simulink model "Modello_Irb1300_R2022a"  (R2022a)
settings: Solver=VariableStepAuto  StartTime=0.0  StopTime=56.0  RelTol=1e-3
undefined symbols (not defined in the file or in its folder): DiscIntNeverNeededParam
libraries: vrlib x3, simulink x1
(part 2 of 2)

== matlab function Modello_Irb1300_R2022a/MATLAB Function6 ==
  data: O_d input; R_error output; R_a input
function R_error = Orientation(O_d,R_a)
% R_a, è la matrice di rotazione ottenuta dalla posa in retroazione 

%R_iniziale, questa matrice è la matrice iniziale (orientzione assoluta) 
%che permette di riferire gli angoli di eulero alla orientazione relativa dell'end effector
R_iniziale = [
    0.0000    0.0000    1.0000 ;
    1.0000         0    0.0000 ;
         0    1.0000    0.0000 ];
% Angolipi di Eulero in radianti
theta = O_d(1);  % Rotazione attorno all'asse x 
phi = O_d(2);    % Rotazione attorno all'asse y 
psi = O_d(3);    % Rotazione attorno all'asse z (psi = 0° otteniamo una rotazione dell'end effector di 90°)

% Matrici di rotazione elementari
R_x = [
      1, 0, 0;
      0, cos(theta), -sin(theta);
      0, sin(theta), cos(theta)
];

R_y = [
    cos(phi), 0, sin(phi);
    0, 1, 0;
    -sin(phi), 0, cos(phi)
];

R_z = [
    cos(psi), -sin(psi), 0;
    sin(psi), cos(psi), 0;
    0, 0, 1
];

% Matrice di rotazione totale
% R_d_rel consiste nella matrice di rotazione desiderate relativa all'endeffector
R_d_rel = R_z * R_y * R_x;  % Ordine: ZYX (dipende dalla convenzione scelta)

%R_d_ass consiste nella matrice di rotazione desiderata assoluta espressa
%rispetto la terna di base del robot 
R_d_ass = R_iniziale * R_d_rel;

R_error = R_d_ass * R_a';

end

% function omega_e = calcOmegaError(R_d, R_a)
%     % Calcola la matrice di errore
%     R_error = R_d * R_a';
% 
%     % Calcola theta
%     theta = acos((trace(R_error) - 1) / 2);
% 
%     % Calcola matrice antisimmetrica u_hat
%     if abs(sin(theta)) > 1e-6  % Evita divisioni per zero
%         u_hat = (R_error - R_error') / (2 * sin(theta));
%     else
%         u_hat = zeros(3);  % Caso limite (errore molto piccolo)
%     end
% 
%     % Estrai omega_e usando vex
%     omega_e = [u_hat(3, 2); u_hat(1, 3); u_hat(2, 1)];
% end
% 
% 






% % Angoli di Eulero in radianti
% theta = pi/6;  % Rotazione attorno all'asse x (30°)
% phi = pi/4;    % Rotazione attorno all'asse y (45°)
% psi = pi/3;    % Rotazione attorno all'asse z (60°)
% 
% % Matrici di rotazione elementari
% R_x = [
%     1, 0, 0;
%     0, cos(theta), -sin(theta);
%     0, sin(theta), cos(theta)
% ];
% R_y = [
%     cos(phi), 0, sin(phi);
%     0, 1, 0;
%     -sin(phi), 0, cos(phi)
% ];
% R_z = [
%     cos(psi), -sin(psi), 0;
%     sin(psi), cos(psi), 0;
%     0, 0, 1
% ];
% 
% % Matrice di rotazione totale
% R_d = R_z * R_y * R_x;  % Ordine: ZYX (dipende dalla convenzione scelta)

% % Inizializzo la matrice che definisce l'orientazione desidarata 
% % In questo esempio, R_d è una matrice di rotazione che rappresenta una rotazione 
% % di 30° rispetto all'asse Z.
% R_d = [0.866, -0.5, 0;
%        0.5,  0.866, 0;
%          0,      0, 1];

== matlab function Modello_Irb1300_R2022a/MATLAB Function7 ==
  data: R_error input; omega output
% function omega = calcAngularVelocity(R_error)
%     omega = 0.5 * [
%         R_error(3,2) - R_error(2,3);
%         R_error(1,3) - R_error(3,1);
%         R_error(2,1) - R_error(1,2)
%     ];
% end

 function omega = calcOmegaError(R_error)
    % Calcola la matrice di errore

    % Calcola theta
    theta = acos((trace(R_error) - 1) / 2);

    % Calcola matrice antisimmetrica u_hat
    if abs(theta) < 1e-6  % Evita divisioni per zero
        omega = [0;0;0];
    else
        skew_matrix = (R_error - R_error')/(2*sin(theta));  % Caso limite (errore molto piccolo)
        omega = [skew_matrix(3,2);skew_matrix(1,3);skew_matrix(2,1)];
    end

    % Estrai omega_e usando vex
    omega = theta * omega;
end
